simulink model "Final_Model_origin"  (R2022b)
settings: Solver=VariableStepAuto  StartTime=0.0  StopTime=3600 * 3  RelTol=1e-3  AbsTol=1e-3
InitFcn:
  | RT_env = 30; % [degC] External environment temperature
  | RH_env = 0.5; % External environment relative humidity
  | 
  | RH_house_init = 0.5; % Initial house relative humidity
  | 
  | tube_D = 0.02; % [m] Refrigerant tube diameter
  | duct_W = 0.4; % [m] Air duct width
  | 
  | house_L = 20; % [m] House length
  | house_W = 10; % [m] House width
  | house_H = 6; % [m] House height
  | roof_pitch = 40; % [deg] Roof pitch
  | A_I
  | A_IV
  | A_VIII
  | A_V
  | B_II
  | A_II
  | A_VI
undefined symbols (not defined in the file or in its folder): alpha_h_ratio, area_furniture, area_roof, area_wall_exterior, area_window, cp_furniture, cp_roof, cp_wall_exterior, cp_window, hc_furniture_interior, hc_roof_exterior, hc_roof_interior, hc_wall_exterior, hc_wall_interior, hc_window_exterior, hc_window_interior, k_roof, k_wall, k_window, l_roof, mass_furniture, no_motors, no_occupants, pitch_roof, Q_infiltration, Q_latent_occupant_skin, Q_lights, Q_occupant, rho_roof, rho_wall, rho_window, SC, sigbuilder_block, T_house_init, T_init_furniture, T_set, thicnkess_roof, thicnkess_wall_exterior, thicnkess_window, U_roof, U_wall, U_window, w_roof
libraries: fl_lib x81, nesl_utility x24, SimscapeFluids_lib x9, simulink_extras x3
(part 3 of 3)

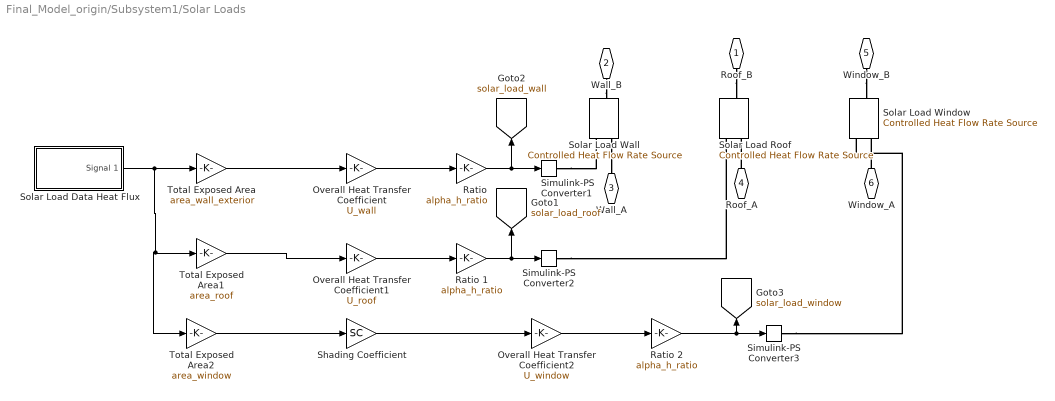
== system Final_Model_origin/Subsystem1/Solar Loads ==
  Overall Heat Transfer Coefficient : Gain  Gain=U_wall
  Overall Heat Transfer Coefficient1 : Gain  Gain=U_roof
  Overall Heat Transfer Coefficient2 : Gain  Gain=U_window
  "Ratio " : Gain  Gain=alpha_h_ratio
  Ratio 1 : Gain  Gain=alpha_h_ratio
  Ratio 2 : Gain  Gain=alpha_h_ratio
  Shading Coefficient : Gain  Gain=SC
  Simulink-PS Converter1 : nesl_utility/Simulink-PS Converter  PhysicalDomain=network_engine_domain  SubClassName=ps_input  LeftPortType=input  RightPortType=output  PseudoPeriodic=off  Frequencies=[]  NoiseDistribution=none  NoiseParameters=[]  Unit=1  AffineConversion=off  FilteringAndDerivatives=provide  SimscapeFilterOrder=1  InputFilterTimeConstant=0.001  UdotUserProvided=0
  Simulink-PS Converter2 : nesl_utility/Simulink-PS Converter  PhysicalDomain=network_engine_domain  SubClassName=ps_input  LeftPortType=input  RightPortType=output  PseudoPeriodic=off  Frequencies=[]  NoiseDistribution=none  NoiseParameters=[]  Unit=1  AffineConversion=off  FilteringAndDerivatives=provide  SimscapeFilterOrder=1  InputFilterTimeConstant=0.001  UdotUserProvided=0
  Simulink-PS Converter3 : nesl_utility/Simulink-PS Converter  PhysicalDomain=network_engine_domain  SubClassName=ps_input  LeftPortType=input  RightPortType=output  PseudoPeriodic=off  Frequencies=[]  NoiseDistribution=none  NoiseParameters=[]  Unit=1  AffineConversion=off  FilteringAndDerivatives=provide  SimscapeFilterOrder=1  InputFilterTimeConstant=0.001  UdotUserProvided=0
  Solar Load Data Heat Flux : Subsystem  Tag=STV Subsys  LoadFcn=sigbuilder_block('load');  StartFcn=sigbuilder_block('start');  StopFcn=sigbuilder_block('stop');  ClipboardFcn=sigbuilder_block('clipboard');  mask(Sigbuilder block){tuvar=[0:10]}
      mask help: Simulink:masks:SigbuilderBlock_MD
      mask init:
      | if ~strcmp(get_param(bdroot(gcbh),'SimulationStatus'),'stopped') tuvar = sigbuilder_block('maskInit'); end
      settings: CopyFcn=sigbuilder_block('copy');  DeleteFcn=sigbuilder_block('delete');  ModelCloseFcn=sigbuilder_block('modelClose');  PreSaveFcn=sigbuilder_block('preSave');  PauseFcn=sigbuilder_block('pause');  ContinueFcn=sigbuilder_block('continue');  NameChangeFcn=sigbuilder_block('namechange');  OpenFcn=sigbuilder_block('open',[440 197.091 394.909 397.818 ]);  CloseFcn=sigbuilder_block('close');
      mask Display: plot(0, 0, 100, 100,[2, 2, 32, 32, 2], [68, 8, 8, 68, 68],[32, 2], [38, 38], [32, 19, 2],[53, 60, 44], [32, 17, 17, 2],[16, 16, 31, 31]);txt = getActiveGroup(gcbh);text(2, 100, txt,'verticalAlignment', 'top');
  Solar Load Roof : fl_lib/Thermal/Thermal Sources/Controlled Heat Flow Rate Source
  Solar Load Wall : fl_lib/Thermal/Thermal Sources/Controlled Heat Flow Rate Source
  Solar Load Window : fl_lib/Thermal/Thermal Sources/Controlled Heat Flow Rate Source
  Total Exposed Area : Gain  Gain=area_wall_exterior
  Total Exposed Area1 : Gain  Gain=area_roof
  Total Exposed Area2 : Gain  Gain=area_window
  Roof_B : PMIOPort  Side=Left
  Wall_B : PMIOPort  Port=2  Side=Left
  Wall_A : PMIOPort  Port=3  Side=Right
  Roof_A : PMIOPort  Port=4  Side=Right
  Window_B : PMIOPort  Port=5  Side=Right
  Window_A : PMIOPort  Port=6  Side=Right
  tag scope: solar_load_roof=global, solar_load_wall=global, solar_load_window=global
  wires:
  "Ratio "/1 -> [solar_load_wall], Simulink-PS Converter1/1
  Solar Load Data Heat Flux/1(Signal 1) -> Total Exposed Area1/1, Total Exposed Area2/1, Total Exposed Area/1
  Total Exposed Area/1 -> Overall Heat Transfer Coefficient/1
  Overall Heat Transfer Coefficient/1 -> "Ratio "/1
  Total Exposed Area1/1 -> Overall Heat Transfer Coefficient1/1
  Overall Heat Transfer Coefficient1/1 -> Ratio 1/1
  Ratio 1/1 -> [solar_load_roof], Simulink-PS Converter2/1
  Overall Heat Transfer Coefficient2/1 -> Ratio 2/1
  Ratio 2/1 -> [solar_load_window], Simulink-PS Converter3/1
  Total Exposed Area2/1 -> Shading Coefficient/1
  Shading Coefficient/1 -> Overall Heat Transfer Coefficient2/1
  connections:
  Simulink-PS Converter1/RConn1 -- Solar Load Wall/RConn1
  Simulink-PS Converter2/RConn1 -- Solar Load Roof/RConn1
  Simulink-PS Converter3/RConn1 -- Solar Load Window/RConn1
  Wall_B/RConn1 -- Solar Load Wall/LConn1
  Solar Load Wall/RConn2 -- Wall_A/RConn1
  Window_A/RConn1 -- Solar Load Window/RConn2
  Window_B/RConn1 -- Solar Load Window/LConn1
  Roof_B/RConn1 -- Solar Load Roof/LConn1
  Roof_A/RConn1 -- Solar Load Roof/RConn2

== system Final_Model_origin/Subsystem1/Solar Loads/Solar Load Data Heat Flux ==
  Demux : Demux  Tag=STV Demux  Outputs=1
      settings: DisplayOption=none
  FromWs : FromWorkspace  Tag=STV FromWs  VariableName=tuvar
      SigBuilderData=|
      | common.afterFinalStr = 'Extrapolate'
      | common.sampleTime = 0
      | dataSet.timeRange = [0 32400]
      | dataSet.name = 'Group 1'
      | sbobj.Groups.Name = 'Group 1'
      | sbobj.Groups.Signals.Name = 'Signal 1'
      | sbobj.Groups.Signals.XData = [0 3600 7200 10800 14400 18000 21600 25200 28800 32400]
      | sbobj.Groups.Signals.YData = [483 811 875 803 647 428 185 48 20 0]
      | sbobj.Groups.TimeRange = [0 32400]
  Signal 1 : Outport  Tag=STV Outport
  wires:
  Demux/1 -> Signal 1/1
  FromWs/1 -> Demux/1
